simulink model "ploop_test_modify2017"  (R2017a)
settings: Solver=FixedStepAuto  StartTime=0.0  StopTime=Tf  FixedStep=delta_r  RelTol=1e-3  EnableMultiTasking=on
values from neighbouring files (symbols this model uses):
  delta_r = 1/500    (= 0.002)    [p560_simulation_main_position.m]
  delta_t = 1/500    (= 0.002)    [p560_simulation_main_position.m]
  Kd = 0.0006    [p560_simulation_main_position.m]
  Kg = 1/107.815    (= 0.00927514724296)    [p560_simulation_main_position.m]
  Q = 30    [p560_simulation_main_position.m]
  q0 = q0_m(yh)    [p560_simulation_main_position.m]
  R = 3    [p560_simulation_main_position.m]
  S = 600    [p560_simulation_main_position.m]
  time_delay = 0    [p560_simulation_main_position.m]
undefined symbols (not defined in the file or in its folder): time_delayp, yh
libraries: sldrtlib x1
settings Model: Creator=pic  LastModifiedBy=yehanspc
settings DataIOCC: SaveFormat=Array  SignalLoggingSaveFormat=ModelDataLogs  ReturnWorkspaceOutputs=on  TimeSaveName=t  OutputSaveName=y  OutputOption=SpecifiedOutputTimes  OutputTimes=[0:0.001:1]'
settings OptimizationCC: ExpressionDepthLimit=2147483647  LifeSpan=inf
settings DebuggingCC: UnderspecifiedInitializationDetection=Classic  MergeDetectMultiDrivingBlocksExec=none  SolverPrmCheckMsg=warning  AllowSymbolicDim=off  StateNameClashWarn=warning  SFUnexpectedBacktrackingDiag=warning  SFNoUnconditionalDefaultTransitionDiag=warning  SFExecutionAtInitializationDiag=none
settings HardwareCC: ProdBitPerPointer=32  ProdBitPerSizeT=32  ProdBitPerPtrDiffT=32  ProdLargestAtomicFloat=None  ProdIntDivRoundTo=Undefined  ProdEndianess=Unspecified  ProdWordSize=32  ProdHWDeviceType=32-bit Generic
settings ModelReferenceCC: PropagateSignalLabelsOutOfModel=off
settings GRTTargetCC: TargetLangStandard=C89/C90 (ANSI)  GeneratePreprocessorConditionals=Disable all  CombineOutputUpdateFcns=off  GRTInterface=on
settings ConfigComp: CovMetricSettings=dw  CovHtmlReporting=on  CovSaveCumulativeToWorkspaceVar=on  CovSaveSingleToWorkspaceVar=on  CovExternalEMLEnable=off  CovSFcnEnable=off

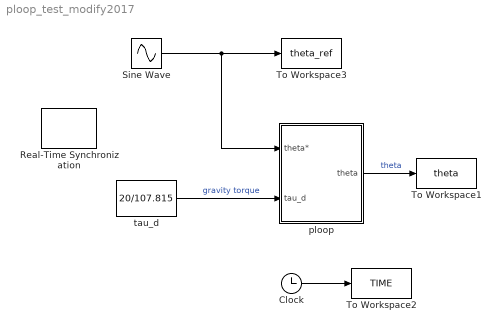
== system ploop_test_modify2017 ==
  Clock : Clock
  Real-Time Synchronization : sldrtlib/Real-Time Synchronization  SampleTime=delta_r  MaxMissedTicks=10000  ShowMissedTicks=off  YieldWhenWaiting=off
  Sine Wave : Sin  Amplitude=6  Frequency=1.2  Phase=pi/2  SampleTime=0
  To Workspace1 : ToWorkspace  VariableName=theta  SaveFormat=Timeseries  SampleTime=-1
  To Workspace2 : ToWorkspace  VariableName=TIME  SaveFormat=Timeseries  SampleTime=-1
  To Workspace3 : ToWorkspace  VariableName=theta_ref  SaveFormat=Timeseries  SampleTime=-1
  ploop : Subsystem
  tau_d : Constant  Value=20/107.815
  wires:
  ploop/1(theta) -> To Workspace1/1  "theta"
  Sine Wave/1 -> ploop/1(theta*), To Workspace3/1
  tau_d/1 -> ploop/2(tau_d)  "gravity torque"
  Clock/1 -> To Workspace2/1

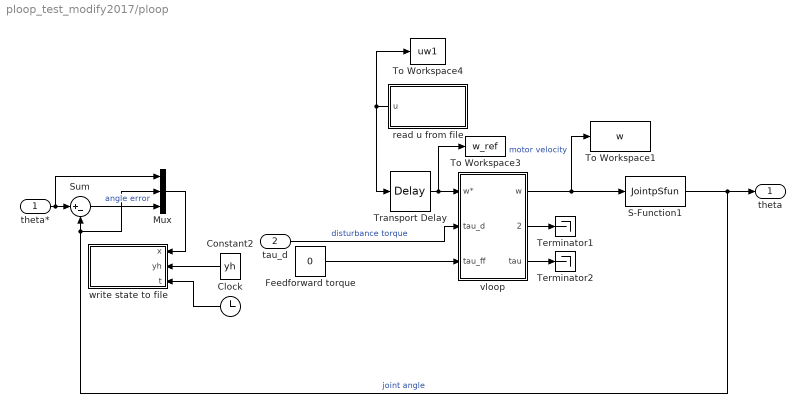
== system ploop_test_modify2017/ploop ==
  theta* : Inport
  tau_d : Inport  Port=2
  Clock : Clock
  Constant2 : Constant  Value=yh
  Feedforward torque : Constant  Value=0
  Mux : Mux  Inputs=3
  S-Function1 : S-Function  FunctionName=JointpSfun  Parameters=Kg,delta_r,q0  SFunctionDeploymentMode=off  EnableBusSupport=off
  Sum : Sum  Inputs=|+-
  Terminator1 : Terminator
  Terminator2 : Terminator
  To Workspace1 : ToWorkspace  VariableName=w  SaveFormat=Timeseries  SampleTime=-1
  To Workspace3 : ToWorkspace  VariableName=w_ref  SaveFormat=Timeseries  SampleTime=-1
  To Workspace4 : ToWorkspace  VariableName=uw1  SaveFormat=Timeseries  SampleTime=-1
  Transport Delay : TransportDelay  DelayTime=time_delayp
  read u from file : MATLAB Function  TreatAsAtomicUnit=on
  vloop : Subsystem  AncestorBlock=roblocks/Arm/vloop  mask{J=580e-6, B=817e-6, Km=0.228, tau_max=0.9, Kv=1, Ki=0, T=0.001}
      mask prompts: J "Inertia (J)"; B "Viscous friction coefficient (B)"; Km "Motor torque constant"; tau_max "Torque limit (tau_max)"; Kv "Proportional gain (Kv)"; Ki "Integral gain (Ki)"; T "Sample interval (T)"
  write state to file : MATLAB Function  TreatAsAtomicUnit=on
  theta : Outport
  wires:
  Sum/1 -> Mux/3  "angle error"
  S-Function1/1 -> theta/1, Mux/2, Sum/2  "joint angle"
  theta*/1 -> Mux/1, Sum/1
  vloop/2(w error) -> Terminator1/1
  vloop/3(tau) -> Terminator2/1
  vloop/1(w) -> S-Function1/1, To Workspace1/1  "motor velocity"
  tau_d/1 -> vloop/2(tau_d)  "disturbance torque"
  Feedforward torque/1 -> vloop/3(tau_ff)
  Transport Delay/1 -> vloop/1(w*), To Workspace3/1
  Constant2/1 -> write state to file/2(yh)
  Mux/1 -> write state to file/1(x)
  read u from file/1(u) -> Transport Delay/1, To Workspace4/1
  Clock/1 -> write state to file/3(t)

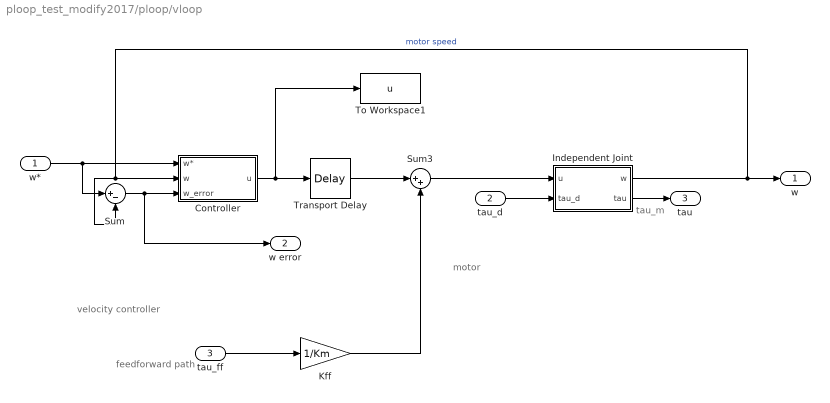
== system ploop_test_modify2017/ploop/vloop ==
  note: velocity controller
  note: feedforward path
  note: tau_m
  note: motor
  w* : Inport
  tau_d : Inport  Port=2
  tau_ff : Inport  Port=3
  Controller : Subsystem
  Independent Joint : Subsystem
  Kff : Gain  Gain=1/Km
  Sum : Sum  Inputs=|+-
  Sum3 : Sum  Inputs=|++
  To Workspace1 : ToWorkspace  VariableName=u  SaveFormat=Timeseries  SampleTime=-1
  Transport Delay : TransportDelay  DelayTime=time_delay
  w : Outport
  w error : Outport  Port=2
  tau : Outport  Port=3
  wires:
  tau_ff/1 -> Kff/1
  Kff/1 -> Sum3/2
  Sum3/1 -> Independent Joint/1(u)
  tau_d/1 -> Independent Joint/2(tau_d)
  Independent Joint/1(w) -> Sum/2, Controller/2(w), w/1  "motor speed"
  w*/1 -> Sum/1, Controller/1(w*)
  Sum/1 -> w error/1, Controller/3(w_error)
  Transport Delay/1 -> Sum3/1
  Controller/1(u) -> Transport Delay/1, To Workspace1/1
  Independent Joint/2(tau) -> tau/1

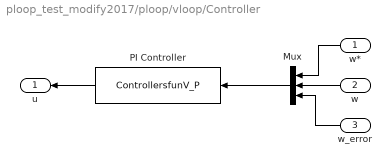
== system ploop_test_modify2017/ploop/vloop/Controller ==
  w* : Inport
  w : Inport  Port=2
  w_error : Inport  Port=3
  Mux : Mux  Inputs=3
  PI Controller : S-Function  FunctionName=ControllersfunV_P  Parameters=Kv,Ki,Kd,delta_t,delta_r,B,J,Km,Q,R,S  SFunctionDeploymentMode=off  EnableBusSupport=off
  u : Outport
  wires:
  w/1 -> Mux/2
  w*/1 -> Mux/1
  Mux/1 -> PI Controller/1
  PI Controller/1 -> u/1
  w_error/1 -> Mux/3

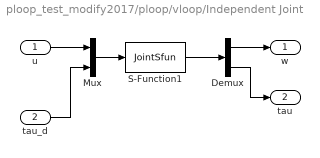
== system ploop_test_modify2017/ploop/vloop/Independent Joint ==
  u : Inport
  tau_d : Inport  Port=2
  Demux : Demux  Outputs=2
  Mux : Mux  Inputs=2
  S-Function1 : S-Function  FunctionName=JointSfun  Parameters=B,J,Km,delta_r  SFunctionDeploymentMode=off  EnableBusSupport=off
  w : Outport
  tau : Outport  Port=2
  wires:
  Mux/1 -> S-Function1/1
  u/1 -> Mux/1
  tau_d/1 -> Mux/2
  S-Function1/1 -> Demux/1
  Demux/1 -> w/1
  Demux/2 -> tau/1

== matlab function ploop_test_modify2017/ploop/write state to file ==
  data: x input; yh input; t input
function write_block(x,yh,t)
% Inputs:
% ymea: measurement from structure
% Outputs:
% ymea1: measurement output

eml.extrinsic('write_x');
write_x(x,yh,t);

== matlab function ploop_test_modify2017/ploop/read u from file ==
  data: u output
function u = read_u_block
% Inputs:
% ymea: measurement from structure
% Outputs:
% ymea1: measurement output

% coder.extrinsic('fscanf')
u=0;
eml.extrinsic('read_u');
% 
u = read_u();
